simulink model "PannelTest"  (R2022b)
settings: Solver=FixedStepAuto  StartTime=0.0  StopTime=102  FixedStep=0.001  RelTol=1e-3
model workspace (MAT data in the model file):
  Manual_Auto : Simulink.Parameter (value not decoded)
  Pattern : Simulink.Parameter (value not decoded)
  Pause_Start : Simulink.Parameter (value not decoded)
  Stop : Simulink.Parameter (value not decoded)
  Unlock_Lock : Simulink.Parameter (value not decoded)
undefined symbols (not defined in the file or in its folder): DiscIntNeverNeededParam
(part 2 of 3)

== system PannelTest/PanelController/Display_State_4_Enable/Subsystem ==
  Case : Inport
  Case Default : Inport  Port=2
  Constant : Constant
  Constant1 : Constant  Value=0
  Constant2 : Constant  Value=TaskIndex
  Merge : Merge
  Switch Case Action Subsystem : Subsystem  TreatAsAtomicUnit=on
  Switch Case Action Subsystem1 : Subsystem  TreatAsAtomicUnit=on
  Enable : Outport
  FinishIndex : Outport  Port=2
  wires:
  Constant/1 -> Switch Case Action Subsystem/1(In1)
  Case/1 -> Switch Case Action Subsystem/Action
  Switch Case Action Subsystem/1(Out1) -> Merge/1
  Merge/1 -> Enable/1
  Case Default/1 -> Switch Case Action Subsystem1/Action
  Constant1/1 -> Switch Case Action Subsystem1/1(In1)
  Switch Case Action Subsystem1/1(Default) -> Merge/2
  Constant2/1 -> FinishIndex/1

== system PannelTest/PanelController/LLTaskControl_State_1_Enable/Subsystem ==
  Case : Inport
  Case Default : Inport  Port=2
  Constant : Constant
  Constant1 : Constant  Value=0
  Constant2 : Constant  Value=TaskIndex
  Merge : Merge
  Switch Case Action Subsystem : Subsystem  TreatAsAtomicUnit=on
  Switch Case Action Subsystem1 : Subsystem  TreatAsAtomicUnit=on
  Enable : Outport
  FinishIndex : Outport  Port=2
  wires:
  Constant/1 -> Switch Case Action Subsystem/1(In1)
  Case/1 -> Switch Case Action Subsystem/Action
  Switch Case Action Subsystem/1(Out1) -> Merge/1
  Merge/1 -> Enable/1
  Case Default/1 -> Switch Case Action Subsystem1/Action
  Constant1/1 -> Switch Case Action Subsystem1/1(In1)
  Switch Case Action Subsystem1/1(Default) -> Merge/2
  Constant2/1 -> FinishIndex/1

== system PannelTest/PanelController/LLTaskControl_State_2_Enable/Subsystem ==
  Case : Inport
  Case Default : Inport  Port=2
  Constant : Constant
  Constant1 : Constant  Value=0
  Constant2 : Constant  Value=TaskIndex
  Merge : Merge
  Switch Case Action Subsystem : Subsystem  TreatAsAtomicUnit=on
  Switch Case Action Subsystem1 : Subsystem  TreatAsAtomicUnit=on
  Enable : Outport
  FinishIndex : Outport  Port=2
  wires:
  Constant/1 -> Switch Case Action Subsystem/1(In1)
  Case/1 -> Switch Case Action Subsystem/Action
  Switch Case Action Subsystem/1(Out1) -> Merge/1
  Merge/1 -> Enable/1
  Case Default/1 -> Switch Case Action Subsystem1/Action
  Constant1/1 -> Switch Case Action Subsystem1/1(In1)
  Switch Case Action Subsystem1/1(Default) -> Merge/2
  Constant2/1 -> FinishIndex/1

== system PannelTest/PanelController/LLTaskControl_State_3_Enable/Subsystem ==
  Case : Inport
  Case Default : Inport  Port=2
  Constant : Constant
  Constant1 : Constant  Value=0
  Constant2 : Constant  Value=TaskIndex
  Merge : Merge
  Switch Case Action Subsystem : Subsystem  TreatAsAtomicUnit=on
  Switch Case Action Subsystem1 : Subsystem  TreatAsAtomicUnit=on
  Enable : Outport
  FinishIndex : Outport  Port=2
  wires:
  Constant/1 -> Switch Case Action Subsystem/1(In1)
  Case/1 -> Switch Case Action Subsystem/Action
  Switch Case Action Subsystem/1(Out1) -> Merge/1
  Merge/1 -> Enable/1
  Case Default/1 -> Switch Case Action Subsystem1/Action
  Constant1/1 -> Switch Case Action Subsystem1/1(In1)
  Switch Case Action Subsystem1/1(Default) -> Merge/2
  Constant2/1 -> FinishIndex/1

== system PannelTest/PanelController/LLTaskControl_State_4_Enable/Subsystem ==
  Case : Inport
  Case Default : Inport  Port=2
  Constant : Constant
  Constant1 : Constant  Value=0
  Constant2 : Constant  Value=TaskIndex
  Merge : Merge
  Switch Case Action Subsystem : Subsystem  TreatAsAtomicUnit=on
  Switch Case Action Subsystem1 : Subsystem  TreatAsAtomicUnit=on
  Enable : Outport
  FinishIndex : Outport  Port=2
  wires:
  Constant/1 -> Switch Case Action Subsystem/1(In1)
  Case/1 -> Switch Case Action Subsystem/Action
  Switch Case Action Subsystem/1(Out1) -> Merge/1
  Merge/1 -> Enable/1
  Case Default/1 -> Switch Case Action Subsystem1/Action
  Constant1/1 -> Switch Case Action Subsystem1/1(In1)
  Switch Case Action Subsystem1/1(Default) -> Merge/2
  Constant2/1 -> FinishIndex/1

== system PannelTest/PanelController/LLTaskControl_State_5_Enable/Subsystem ==
  Case : Inport
  Case Default : Inport  Port=2
  Constant : Constant
  Constant1 : Constant  Value=0
  Constant2 : Constant  Value=TaskIndex
  Merge : Merge
  Switch Case Action Subsystem : Subsystem  TreatAsAtomicUnit=on
  Switch Case Action Subsystem1 : Subsystem  TreatAsAtomicUnit=on
  Enable : Outport
  FinishIndex : Outport  Port=2
  wires:
  Constant/1 -> Switch Case Action Subsystem/1(In1)
  Case/1 -> Switch Case Action Subsystem/Action
  Switch Case Action Subsystem/1(Out1) -> Merge/1
  Merge/1 -> Enable/1
  Case Default/1 -> Switch Case Action Subsystem1/Action
  Constant1/1 -> Switch Case Action Subsystem1/1(In1)
  Switch Case Action Subsystem1/1(Default) -> Merge/2
  Constant2/1 -> FinishIndex/1

== system PannelTest/PanelController/LLTaskControl_State_6_Enable/Subsystem ==
  Case : Inport
  Case Default : Inport  Port=2
  Constant : Constant
  Constant1 : Constant  Value=0
  Constant2 : Constant  Value=TaskIndex
  Merge : Merge
  Switch Case Action Subsystem : Subsystem  TreatAsAtomicUnit=on
  Switch Case Action Subsystem1 : Subsystem  TreatAsAtomicUnit=on
  Enable : Outport
  FinishIndex : Outport  Port=2
  wires:
  Constant/1 -> Switch Case Action Subsystem/1(In1)
  Case/1 -> Switch Case Action Subsystem/Action
  Switch Case Action Subsystem/1(Out1) -> Merge/1
  Merge/1 -> Enable/1
  Case Default/1 -> Switch Case Action Subsystem1/Action
  Constant1/1 -> Switch Case Action Subsystem1/1(In1)
  Switch Case Action Subsystem1/1(Default) -> Merge/2
  Constant2/1 -> FinishIndex/1

== system PannelTest/PanelController/LLTaskControl_State_7_Enable/Subsystem ==
  Case : Inport
  Case Default : Inport  Port=2
  Constant : Constant
  Constant1 : Constant  Value=0
  Constant2 : Constant  Value=TaskIndex
  Merge : Merge
  Switch Case Action Subsystem : Subsystem  TreatAsAtomicUnit=on
  Switch Case Action Subsystem1 : Subsystem  TreatAsAtomicUnit=on
  Enable : Outport
  FinishIndex : Outport  Port=2
  wires:
  Constant/1 -> Switch Case Action Subsystem/1(In1)
  Case/1 -> Switch Case Action Subsystem/Action
  Switch Case Action Subsystem/1(Out1) -> Merge/1
  Merge/1 -> Enable/1
  Case Default/1 -> Switch Case Action Subsystem1/Action
  Constant1/1 -> Switch Case Action Subsystem1/1(In1)
  Switch Case Action Subsystem1/1(Default) -> Merge/2
  Constant2/1 -> FinishIndex/1

== system PannelTest/PanelController/LLTaskControl_State_8_Enable/Subsystem ==
  Case : Inport
  Case Default : Inport  Port=2
  Constant : Constant
  Constant1 : Constant  Value=0
  Constant2 : Constant  Value=TaskIndex
  Merge : Merge
  Switch Case Action Subsystem : Subsystem  TreatAsAtomicUnit=on
  Switch Case Action Subsystem1 : Subsystem  TreatAsAtomicUnit=on
  Enable : Outport
  FinishIndex : Outport  Port=2
  wires:
  Constant/1 -> Switch Case Action Subsystem/1(In1)
  Case/1 -> Switch Case Action Subsystem/Action
  Switch Case Action Subsystem/1(Out1) -> Merge/1
  Merge/1 -> Enable/1
  Case Default/1 -> Switch Case Action Subsystem1/Action
  Constant1/1 -> Switch Case Action Subsystem1/1(In1)
  Switch Case Action Subsystem1/1(Default) -> Merge/2
  Constant2/1 -> FinishIndex/1

== system PannelTest/PanelController/LLTaskControl_State_9_Enable/Subsystem ==
  Case : Inport
  Case Default : Inport  Port=2
  Constant : Constant
  Constant1 : Constant  Value=0
  Constant2 : Constant  Value=TaskIndex
  Merge : Merge
  Switch Case Action Subsystem : Subsystem  TreatAsAtomicUnit=on
  Switch Case Action Subsystem1 : Subsystem  TreatAsAtomicUnit=on
  Enable : Outport
  FinishIndex : Outport  Port=2
  wires:
  Constant/1 -> Switch Case Action Subsystem/1(In1)
  Case/1 -> Switch Case Action Subsystem/Action
  Switch Case Action Subsystem/1(Out1) -> Merge/1
  Merge/1 -> Enable/1
  Case Default/1 -> Switch Case Action Subsystem1/Action
  Constant1/1 -> Switch Case Action Subsystem1/1(In1)
  Switch Case Action Subsystem1/1(Default) -> Merge/2
  Constant2/1 -> FinishIndex/1

== system PannelTest/PanelController/ULTaskControl_State_1_Enable/Subsystem ==
  Case : Inport
  Case Default : Inport  Port=2
  Constant : Constant
  Constant1 : Constant  Value=0
  Constant2 : Constant  Value=TaskIndex
  Merge : Merge
  Switch Case Action Subsystem : Subsystem  TreatAsAtomicUnit=on
  Switch Case Action Subsystem1 : Subsystem  TreatAsAtomicUnit=on
  Enable : Outport
  FinishIndex : Outport  Port=2
  wires:
  Constant/1 -> Switch Case Action Subsystem/1(In1)
  Case/1 -> Switch Case Action Subsystem/Action
  Switch Case Action Subsystem/1(Out1) -> Merge/1
  Merge/1 -> Enable/1
  Case Default/1 -> Switch Case Action Subsystem1/Action
  Constant1/1 -> Switch Case Action Subsystem1/1(In1)
  Switch Case Action Subsystem1/1(Default) -> Merge/2
  Constant2/1 -> FinishIndex/1

== system PannelTest/PanelController/ULTaskControl_State_2_Enable/Subsystem ==
  Case : Inport
  Case Default : Inport  Port=2
  Constant : Constant
  Constant1 : Constant  Value=0
  Constant2 : Constant  Value=TaskIndex
  Merge : Merge
  Switch Case Action Subsystem : Subsystem  TreatAsAtomicUnit=on
  Switch Case Action Subsystem1 : Subsystem  TreatAsAtomicUnit=on
  Enable : Outport
  FinishIndex : Outport  Port=2
  wires:
  Constant/1 -> Switch Case Action Subsystem/1(In1)
  Case/1 -> Switch Case Action Subsystem/Action
  Switch Case Action Subsystem/1(Out1) -> Merge/1
  Merge/1 -> Enable/1
  Case Default/1 -> Switch Case Action Subsystem1/Action
  Constant1/1 -> Switch Case Action Subsystem1/1(In1)
  Switch Case Action Subsystem1/1(Default) -> Merge/2
  Constant2/1 -> FinishIndex/1

== system PannelTest/Tasks/LLBAutoTask/If Action Subsystem12 ==
  In1 : Inport
  Action Port : ActionPort  ActionPortLabel=if((u1 > 4))
  Out1 : Outport
  wires:
  In1/1 -> Out1/1

== system PannelTest/Tasks/LLBAutoTask/If Action Subsystem13 ==
  In1 : Inport
  Action Port : ActionPort  ActionPortLabel=else
  Out1 : Outport
  wires:
  In1/1 -> Out1/1

== system PannelTest/Tasks/LLBManualTask/If Action Subsystem12 ==
  In1 : Inport
  Action Port : ActionPort  ActionPortLabel=if((u1 > 4))
  Out1 : Outport
  wires:
  In1/1 -> Out1/1

== system PannelTest/Tasks/LLBManualTask/If Action Subsystem13 ==
  In1 : Inport
  Action Port : ActionPort  ActionPortLabel=else
  Out1 : Outport
  wires:
  In1/1 -> Out1/1

== system PannelTest/Tasks/LLFKAutoTask/If Action Subsystem12 ==
  In1 : Inport
  Action Port : ActionPort  ActionPortLabel=if((u1 > 4))
  Out1 : Outport
  wires:
  In1/1 -> Out1/1

== system PannelTest/Tasks/LLFKAutoTask/If Action Subsystem13 ==
  In1 : Inport
  Action Port : ActionPort  ActionPortLabel=else
  Out1 : Outport
  wires:
  In1/1 -> Out1/1

== system PannelTest/Tasks/LLFKManualTask/If Action Subsystem12 ==
  In1 : Inport
  Action Port : ActionPort  ActionPortLabel=if((u1 > 4))
  Out1 : Outport
  wires:
  In1/1 -> Out1/1

== system PannelTest/Tasks/LLFKManualTask/If Action Subsystem13 ==
  In1 : Inport
  Action Port : ActionPort  ActionPortLabel=else
  Out1 : Outport
  wires:
  In1/1 -> Out1/1

== system PannelTest/Tasks/LLFTask/If Action Subsystem12 ==
  In1 : Inport
  Action Port : ActionPort  ActionPortLabel=if((u1 > 4))
  Out1 : Outport
  wires:
  In1/1 -> Out1/1

== system PannelTest/Tasks/LLFTask/If Action Subsystem13 ==
  In1 : Inport
  Action Port : ActionPort  ActionPortLabel=else
  Out1 : Outport
  wires:
  In1/1 -> Out1/1

== system PannelTest/Tasks/LLWAutoTask/If Action Subsystem12 ==
  In1 : Inport
  Action Port : ActionPort  ActionPortLabel=if((u1 > 4))
  Out1 : Outport
  wires:
  In1/1 -> Out1/1

== system PannelTest/Tasks/LLWAutoTask/If Action Subsystem13 ==
  In1 : Inport
  Action Port : ActionPort  ActionPortLabel=else
  Out1 : Outport
  wires:
  In1/1 -> Out1/1

== system PannelTest/Tasks/LLWManualTask/If Action Subsystem12 ==
  In1 : Inport
  Action Port : ActionPort  ActionPortLabel=if((u1 > 4))
  Out1 : Outport
  wires:
  In1/1 -> Out1/1

== system PannelTest/Tasks/LLWManualTask/If Action Subsystem13 ==
  In1 : Inport
  Action Port : ActionPort  ActionPortLabel=else
  Out1 : Outport
  wires:
  In1/1 -> Out1/1

== system PannelTest/Tasks/PauseTask/If Action Subsystem12 ==
  In1 : Inport
  Action Port : ActionPort  ActionPortLabel=if((u1 > 4))
  Out1 : Outport
  wires:
  In1/1 -> Out1/1

== system PannelTest/Tasks/PauseTask/If Action Subsystem13 ==
  In1 : Inport
  Action Port : ActionPort  ActionPortLabel=else
  Out1 : Outport
  wires:
  In1/1 -> Out1/1

== system PannelTest/Tasks/StopTask/If Action Subsystem10 ==
  y : Inport
  Action Port : ActionPort  ActionPortLabel=if(u1 < -0)
  Out1 : Outport
  wires:
  y/1 -> Out1/1

== system PannelTest/Tasks/StopTask/If Action Subsystem11 ==
  y : Inport
  Action Port : ActionPort  ActionPortLabel=else
  Out1 : Outport
  wires:
  y/1 -> Out1/1

== system PannelTest/Tasks/StopTask/If Action Subsystem12 ==
  In1 : Inport
  Action Port : ActionPort  ActionPortLabel=if((u1 > 4))
  Out1 : Outport
  wires:
  In1/1 -> Out1/1

== system PannelTest/Tasks/StopTask/If Action Subsystem13 ==
  In1 : Inport
  Action Port : ActionPort  ActionPortLabel=else
  Out1 : Outport
  wires:
  In1/1 -> Out1/1

== system PannelTest/Tasks/StopTask/If Action Subsystem4 ==
  In1 : Inport
  Action Port : ActionPort  ActionPortLabel=if((u1 <= 1))
  Out1 : Outport
  wires:
  In1/1 -> Out1/1

== system PannelTest/Tasks/StopTask/If Action Subsystem5 ==
  In1 : Inport
  Action Port : ActionPort  ActionPortLabel=else
  Out1 : Outport
  wires:
  In1/1 -> Out1/1

== system PannelTest/Tasks/StopTask/If Action Subsystem6 ==
  In1 : Inport
  Action Port : ActionPort  ActionPortLabel=if((u1 <= 1))
  Out1 : Outport
  wires:
  In1/1 -> Out1/1

== system PannelTest/Tasks/StopTask/If Action Subsystem7 ==
  In1 : Inport
  Action Port : ActionPort  ActionPortLabel=else
  Out1 : Outport
  wires:
  In1/1 -> Out1/1

== system PannelTest/Tasks/StopTask/If Action Subsystem8 ==
  y : Inport
  Action Port : ActionPort  ActionPortLabel=if(u1 < -0)
  Out1 : Outport
  wires:
  y/1 -> Out1/1

== system PannelTest/Tasks/StopTask/If Action Subsystem9 ==
  In1 : Inport
  Action Port : ActionPort  ActionPortLabel=else
  Out1 : Outport
  wires:
  In1/1 -> Out1/1

== system PannelTest/Tasks/ULLockTask/If Action Subsystem12 ==
  In1 : Inport
  Action Port : ActionPort  ActionPortLabel=if((u1 > 4))
  Out1 : Outport
  wires:
  In1/1 -> Out1/1

== system PannelTest/Tasks/ULLockTask/If Action Subsystem13 ==
  In1 : Inport
  Action Port : ActionPort  ActionPortLabel=else
  Out1 : Outport
  wires:
  In1/1 -> Out1/1

== system PannelTest/Tasks/ULUnLockTask/If Action Subsystem12 ==
  In1 : Inport
  Action Port : ActionPort  ActionPortLabel=if((u1 > 4))
  Out1 : Outport
  wires:
  In1/1 -> Out1/1

== system PannelTest/Tasks/ULUnLockTask/If Action Subsystem13 ==
  In1 : Inport
  Action Port : ActionPort  ActionPortLabel=else
  Out1 : Outport
  wires:
  In1/1 -> Out1/1

== system PannelTest/PanelController/Display_State_1_Enable/Subsystem/Switch Case Action Subsystem ==
  In1 : Inport
  Action Port : ActionPort  ActionPortLabel=case [ 1 ]:
  Out1 : Outport
  wires:
  In1/1 -> Out1/1

== system PannelTest/PanelController/Display_State_1_Enable/Subsystem/Switch Case Action Subsystem1 ==
  In1 : Inport
  Action Port : ActionPort  ActionPortLabel=default:
  Default : Outport
  wires:
  In1/1 -> Default/1

== system PannelTest/PanelController/Display_State_2_Enable/Subsystem/Switch Case Action Subsystem ==
  In1 : Inport
  Action Port : ActionPort  ActionPortLabel=case [ 2 ]:
  Out1 : Outport
  wires:
  In1/1 -> Out1/1

== system PannelTest/PanelController/Display_State_2_Enable/Subsystem/Switch Case Action Subsystem1 ==
  In1 : Inport
  Action Port : ActionPort  ActionPortLabel=default:
  Default : Outport
  wires:
  In1/1 -> Default/1

== system PannelTest/PanelController/Display_State_3_Enable/Subsystem/Switch Case Action Subsystem ==
  In1 : Inport
  Action Port : ActionPort  ActionPortLabel=case [ 3 ]:
  Out1 : Outport
  wires:
  In1/1 -> Out1/1

== system PannelTest/PanelController/Display_State_3_Enable/Subsystem/Switch Case Action Subsystem1 ==
  In1 : Inport
  Action Port : ActionPort  ActionPortLabel=default:
  Default : Outport
  wires:
  In1/1 -> Default/1

== system PannelTest/PanelController/Display_State_4_Enable/Subsystem/Switch Case Action Subsystem ==
  In1 : Inport
  Action Port : ActionPort  ActionPortLabel=case [ 4 ]:
  Out1 : Outport
  wires:
  In1/1 -> Out1/1

== system PannelTest/PanelController/Display_State_4_Enable/Subsystem/Switch Case Action Subsystem1 ==
  In1 : Inport
  Action Port : ActionPort  ActionPortLabel=default:
  Default : Outport
  wires:
  In1/1 -> Default/1

== system PannelTest/PanelController/LLTaskControl_State_1_Enable/Subsystem/Switch Case Action Subsystem ==
  In1 : Inport
  Action Port : ActionPort  ActionPortLabel=case [ 1 ]:
  Out1 : Outport
  wires:
  In1/1 -> Out1/1

== system PannelTest/PanelController/LLTaskControl_State_1_Enable/Subsystem/Switch Case Action Subsystem1 ==
  In1 : Inport
  Action Port : ActionPort  ActionPortLabel=default:
  Default : Outport
  wires:
  In1/1 -> Default/1

== system PannelTest/PanelController/LLTaskControl_State_2_Enable/Subsystem/Switch Case Action Subsystem ==
  In1 : Inport
  Action Port : ActionPort  ActionPortLabel=case [ 2 ]:
  Out1 : Outport
  wires:
  In1/1 -> Out1/1

== system PannelTest/PanelController/LLTaskControl_State_2_Enable/Subsystem/Switch Case Action Subsystem1 ==
  In1 : Inport
  Action Port : ActionPort  ActionPortLabel=default:
  Default : Outport
  wires:
  In1/1 -> Default/1

== system PannelTest/PanelController/LLTaskControl_State_3_Enable/Subsystem/Switch Case Action Subsystem ==
  In1 : Inport
  Action Port : ActionPort  ActionPortLabel=case [ 3 ]:
  Out1 : Outport
  wires:
  In1/1 -> Out1/1

== system PannelTest/PanelController/LLTaskControl_State_3_Enable/Subsystem/Switch Case Action Subsystem1 ==
  In1 : Inport
  Action Port : ActionPort  ActionPortLabel=default:
  Default : Outport
  wires:
  In1/1 -> Default/1

== system PannelTest/PanelController/LLTaskControl_State_4_Enable/Subsystem/Switch Case Action Subsystem ==
  In1 : Inport
  Action Port : ActionPort  ActionPortLabel=case [ 4 ]:
  Out1 : Outport
  wires:
  In1/1 -> Out1/1

== system PannelTest/PanelController/LLTaskControl_State_4_Enable/Subsystem/Switch Case Action Subsystem1 ==
  In1 : Inport
  Action Port : ActionPort  ActionPortLabel=default:
  Default : Outport
  wires:
  In1/1 -> Default/1

== system PannelTest/PanelController/LLTaskControl_State_5_Enable/Subsystem/Switch Case Action Subsystem ==
  In1 : Inport
  Action Port : ActionPort  ActionPortLabel=case [ 5 ]:
  Out1 : Outport
  wires:
  In1/1 -> Out1/1

== system PannelTest/PanelController/LLTaskControl_State_5_Enable/Subsystem/Switch Case Action Subsystem1 ==
  In1 : Inport
  Action Port : ActionPort  ActionPortLabel=default:
  Default : Outport
  wires:
  In1/1 -> Default/1

== system PannelTest/PanelController/LLTaskControl_State_6_Enable/Subsystem/Switch Case Action Subsystem ==
  In1 : Inport
  Action Port : ActionPort  ActionPortLabel=case [ 6 ]:
  Out1 : Outport
  wires:
  In1/1 -> Out1/1

== system PannelTest/PanelController/LLTaskControl_State_6_Enable/Subsystem/Switch Case Action Subsystem1 ==
  In1 : Inport
  Action Port : ActionPort  ActionPortLabel=default:
  Default : Outport
  wires:
  In1/1 -> Default/1

== system PannelTest/PanelController/LLTaskControl_State_7_Enable/Subsystem/Switch Case Action Subsystem ==
  In1 : Inport
  Action Port : ActionPort  ActionPortLabel=case [ 7 ]:
  Out1 : Outport
  wires:
  In1/1 -> Out1/1

== system PannelTest/PanelController/LLTaskControl_State_7_Enable/Subsystem/Switch Case Action Subsystem1 ==
  In1 : Inport
  Action Port : ActionPort  ActionPortLabel=default:
  Default : Outport
  wires:
  In1/1 -> Default/1

== system PannelTest/PanelController/LLTaskControl_State_8_Enable/Subsystem/Switch Case Action Subsystem ==
  In1 : Inport
  Action Port : ActionPort  ActionPortLabel=case [ 8 ]:
  Out1 : Outport
  wires:
  In1/1 -> Out1/1

== system PannelTest/PanelController/LLTaskControl_State_8_Enable/Subsystem/Switch Case Action Subsystem1 ==
  In1 : Inport
  Action Port : ActionPort  ActionPortLabel=default:
  Default : Outport
  wires:
  In1/1 -> Default/1

== system PannelTest/PanelController/LLTaskControl_State_9_Enable/Subsystem/Switch Case Action Subsystem ==
  In1 : Inport
  Action Port : ActionPort  ActionPortLabel=case [ 9 ]:
  Out1 : Outport
  wires:
  In1/1 -> Out1/1

== system PannelTest/PanelController/LLTaskControl_State_9_Enable/Subsystem/Switch Case Action Subsystem1 ==
  In1 : Inport
  Action Port : ActionPort  ActionPortLabel=default:
  Default : Outport
  wires:
  In1/1 -> Default/1

== system PannelTest/PanelController/ULTaskControl_State_1_Enable/Subsystem/Switch Case Action Subsystem ==
  In1 : Inport
  Action Port : ActionPort  ActionPortLabel=case [ 1 ]:
  Out1 : Outport
  wires:
  In1/1 -> Out1/1

== system PannelTest/PanelController/ULTaskControl_State_1_Enable/Subsystem/Switch Case Action Subsystem1 ==
  In1 : Inport
  Action Port : ActionPort  ActionPortLabel=default:
  Default : Outport
  wires:
  In1/1 -> Default/1

== system PannelTest/PanelController/ULTaskControl_State_2_Enable/Subsystem/Switch Case Action Subsystem ==
  In1 : Inport
  Action Port : ActionPort  ActionPortLabel=case [ 2 ]:
  Out1 : Outport
  wires:
  In1/1 -> Out1/1

== system PannelTest/PanelController/ULTaskControl_State_2_Enable/Subsystem/Switch Case Action Subsystem1 ==
  In1 : Inport
  Action Port : ActionPort  ActionPortLabel=default:
  Default : Outport
  wires:
  In1/1 -> Default/1

== stateflow chart PannelTest/PanelController/LowerLimbTaskControlStateMachine ==
  state PauseTask
    ControlState = 9;
  state StopTask
    ControlState = 1;
  state StartTask
    state Start
    state LLFTask
      ControlState = 2;
    state LLFK
      state LLFK
      state LLFKManualTask
        ControlState = 3;
      state LLFKAutoTask
        ControlState = 4;
      (default) -> StartTask.LLFK.LLFK
      StartTask.LLFK.LLFK -> LLFKManualTask [order 1] : [ManualAuto~="LLFK_Auto"]
      StartTask.LLFK.LLFK -> LLFKAutoTask [order 2] : [ManualAuto=="LLFK_Auto"]
      LLFKManualTask -> StartTask.LLFK.LLFK : [ManualAuto=="LLFK_Auto"]
      LLFKAutoTask -> StartTask.LLFK.LLFK : [ManualAuto~="LLFK_Auto"]
    state LLB
      state LLB
      state LLBManualTask
        ControlState = 5;
      state LLBAutoTask
        ControlState = 6;
      (default) -> StartTask.LLB.LLB
      StartTask.LLB.LLB -> LLBAutoTask [order 2] : [ManualAuto=="LLB_Auto"]
      StartTask.LLB.LLB -> LLBManualTask [order 1] : [ManualAuto~="LLB_Auto"]
      LLBAutoTask -> StartTask.LLB.LLB : [ManualAuto~="LLB_Auto"]
      LLBManualTask -> StartTask.LLB.LLB : [ManualAuto=="LLB_Auto"]
    state LLW
      state LLW
      state LLWManualTask
        ControlState = 7;
      state LLWAutoTask
        ControlState = 8;
      (default) -> StartTask.LLW.LLW
      StartTask.LLW.LLW -> LLWManualTask [order 1] : [ManualAuto~="LLW_Auto"]
      StartTask.LLW.LLW -> LLWAutoTask [order 2] : [ManualAuto=="LLW_Auto"]
      LLWAutoTask -> StartTask.LLW.LLW : [ManualAuto~="LLW_Auto"]
      LLWManualTask -> StartTask.LLW.LLW : [ManualAuto=="LLW_Auto"]
    (default) -> Start
    Start -> LLFTask [order 1] : [Mode=="Lower_Limb_Follow"]
    Start -> StartTask.LLFK [order 2] : [Mode=="Lower_Limb_FlutterKick"]
    Start -> StartTask.LLW [order 4] : [Mode=="Lower_Limb_Walk"]
    StartTask.LLB -> Start : [Mode~="Lower_Limb_Breaststroke"]
    LLFTask -> Start : [Mode~="Lower_Limb_Follow"]
    StartTask.LLFK -> Start : [Mode~="Lower_Limb_FlutterKick"]
    StartTask.LLW -> Start : [Mode~="Lower_Limb_Walk"]
    Start -> StartTask.LLB [order 3] : [Mode=="Lower_Limb_Breaststroke"]
  (default) -> PauseTask
  PauseTask -> StartTask [order 2] : [State=="Start"]
  PauseTask -> StopTask [order 1] : [State=="Stop"]
  StartTask -> PauseTask : [State=="Pause"]
  StopTask -> StartTask : [State=="Start"]
  data: State input; Mode input; ManualAuto input; ControlState output; TaskFinished input

== matlab function PannelTest/Tasks/StopTask/MATLAB Function1 ==
  data: u input; y output; Pos input
function y = Current_P(u, Pos)
y = sign(u)*min(abs(u),abs(Pos)*0.1);

== stateflow chart PannelTest/PanelController/KnobStateMachine ==
  state Start
    kState = "Start";
  state Adjust
    state LLF_Adjust
    state Adjust
      kState = "Adjust";
    state LLFK_Adjust
      state LLFK_Auto
      state LLFK_Adjust
        kState = "LLFK_Adjust";
      state LLFK_Freq_Adjust
        state LLFK_Freq_Adjust
          kState = "LLFK_Freq";
          LLFK_Freq = 0;
          LLFK_Torque_Up = 0;
          LLFK_Torque_Down = 0;
          LLFK_Pos_Up = 0;
          LLFK_Pos_Down = 0;
          LLB_Freq = 0;
          LLB_Torque_Up = 0;
          LLB_Torque_Down = 0;
          LLB_Pos_Up = 0;
          LLB_Pos_Down = 0;
          LLW_Freq = 0;
          LLW_Torque_Up = 0;
          LLW_Torque_Down = 0;
          LLW_Pos_Up = 0;
          LLW_Pos_Down = 0;
          Freq_Up_temp = 0;
          Freq_Down_temp = 0;
        state Freq_Up
          if(Freq_Up==0)
          Freq_Up_temp = 0;
          LLFK_Freq = 1;
          end
        state Freq_Down
          if(Freq_Down==0)
          Freq_Down_temp = 0;
          LLFK_Freq = -1;
          end
        (default) -> Adjust.LLFK_Adjust.LLFK_Freq_Adjust.LLFK_Freq_Adjust
        Adjust.LLFK_Adjust.LLFK_Freq_Adjust.LLFK_Freq_Adjust -> Adjust.LLFK_Adjust.LLFK_Freq_Adjust.Freq_Down [order 2] : [(Freq_Down_temp==0)&&(Freq_Down>0)]{Freq_Down_temp=1;}
        Adjust.LLFK_Adjust.LLFK_Freq_Adjust.LLFK_Freq_Adjust -> Adjust.LLFK_Adjust.LLFK_Freq_Adjust.Freq_Up [order 1] : [(Freq_Up_temp==0)&&(Freq_Up>0)]{Freq_Up_temp=1;}
        Adjust.LLFK_Adjust.LLFK_Freq_Adjust.Freq_Up -> Adjust.LLFK_Adjust.LLFK_Freq_Adjust.LLFK_Freq_Adjust : [Freq_Up_temp == 0]
        Adjust.LLFK_Adjust.LLFK_Freq_Adjust.Freq_Down -> Adjust.LLFK_Adjust.LLFK_Freq_Adjust.LLFK_Freq_Adjust : [Freq_Down_temp == 0]
      state LLFK_Torque_Adjust
        state Negtive_Up
          if(Negtive_Up==0)
          Negtive_Up_temp = 0;
          LLFK_Torque_Down = 1;
          end
        state LLFK_Torque_Adjust
          kState = "LLFK_Torq";
          LLFK_Freq = 0;
          LLFK_Torque_Up = 0;
          LLFK_Torque_Down = 0;
          LLFK_Pos_Up = 0;
          LLFK_Pos_Down = 0;
          LLB_Freq = 0;
          LLB_Torque_Up = 0;
          LLB_Torque_Down = 0;
          LLB_Pos_Up = 0;
          LLB_Pos_Down = 0;
          LLW_Freq = 0;
          LLW_Torque_Up = 0;
          LLW_Torque_Down = 0;
          LLW_Pos_Up = 0;
          LLW_Pos_Down = 0;
          Negtive_Up_temp = 0;
          Negtive_Down_temp = 0;
          Positive_Up_temp = 0;
          Positive_Down_temp = 0;
        state Negtive_Down
          if(Negtive_Down==0)
          Negtive_Down_temp = 0;
          LLFK_Torque_Down = -1;
          end
        state Positive_Up
          if(Positive_Up==0)
          Positive_Up_temp = 0;
          LLFK_Torque_Up = 1;
          end
        state Positive_Down
          if(Positive_Down==0)
          Positive_Down_temp = 0;
          LLFK_Torque_Up = -1;
          end
        (default) -> Adjust.LLFK_Adjust.LLFK_Torque_Adjust.LLFK_Torque_Adjust
        Adjust.LLFK_Adjust.LLFK_Torque_Adjust.LLFK_Torque_Adjust -> Adjust.LLFK_Adjust.LLFK_Torque_Adjust.Negtive_Up [order 4] : [(Negtive_Up_temp==0)&&(Negtive_Up>0)]{Negtive_Up_temp=1;}
        Adjust.LLFK_Adjust.LLFK_Torque_Adjust.LLFK_Torque_Adjust -> Adjust.LLFK_Adjust.LLFK_Torque_Adjust.Negtive_Down [order 2] : [(Negtive_Down_temp==0)&&(Negtive_Down>0)]{Negtive_Down_temp=1;}
        Adjust.LLFK_Adjust.LLFK_Torque_Adjust.Negtive_Down -> Adjust.LLFK_Adjust.LLFK_Torque_Adjust.LLFK_Torque_Adjust : [Negtive_Down_temp == 0]
        Adjust.LLFK_Adjust.LLFK_Torque_Adjust.Negtive_Up -> Adjust.LLFK_Adjust.LLFK_Torque_Adjust.LLFK_Torque_Adjust : [Negtive_Up_temp == 0]
        Adjust.LLFK_Adjust.LLFK_Torque_Adjust.LLFK_Torque_Adjust -> Adjust.LLFK_Adjust.LLFK_Torque_Adjust.Positive_Up [order 3] : [(Positive_Up_temp==0)&&(Positive_Up>0)]{Positive_Up_temp=1;}
        Adjust.LLFK_Adjust.LLFK_Torque_Adjust.LLFK_Torque_Adjust -> Adjust.LLFK_Adjust.LLFK_Torque_Adjust.Positive_Down [order 1] : [(Positive_Down_temp==0)&&(Positive_Down>0)]{Positive_Down_temp=1;}
        Adjust.LLFK_Adjust.LLFK_Torque_Adjust.Positive_Up -> Adjust.LLFK_Adjust.LLFK_Torque_Adjust.LLFK_Torque_Adjust : [Positive_Up_temp == 0]
        Adjust.LLFK_Adjust.LLFK_Torque_Adjust.Positive_Down -> Adjust.LLFK_Adjust.LLFK_Torque_Adjust.LLFK_Torque_Adjust : [Positive_Down_temp == 0]
      state LLFK_Pos_Adjust
        state Negtive_Up
          if(Negtive_Up==0)
          Negtive_Up_temp = 0;
          LLFK_Pos_Down = 1;
          end
        state LLFK_Pos_Adjust
          kState = "LLFK_Pos";
          LLFK_Freq = 0;
          LLFK_Torque_Up = 0;
          LLFK_Torque_Down = 0;
          LLFK_Pos_Up = 0;
          LLFK_Pos_Down = 0;
          LLB_Freq = 0;
          LLB_Torque_Up = 0;
          LLB_Torque_Down = 0;
          LLB_Pos_Up = 0;
          LLB_Pos_Down = 0;
          LLW_Freq = 0;
          LLW_Torque_Up = 0;
          LLW_Torque_Down = 0;
          LLW_Pos_Up = 0;
          LLW_Pos_Down = 0;
          Negtive_Up_temp = 0;
          Negtive_Down_temp = 0;
          Positive_Up_temp = 0;
          Positive_Down_temp = 0;
        state Negtive_Down
          if(Negtive_Down==0)
          Negtive_Down_temp = 0;
          LLFK_Pos_Down = -1;
          end
        state Positive_Up
          if(Positive_Up==0)
          Positive_Up_temp = 0;
          LLFK_Pos_Up = 1;
          end
        state Positive_Down
          if(Positive_Down==0)
          Positive_Down_temp = 0;
          LLFK_Pos_Up = -1;
          end
        (default) -> Adjust.LLFK_Adjust.LLFK_Pos_Adjust.LLFK_Pos_Adjust
        Adjust.LLFK_Adjust.LLFK_Pos_Adjust.LLFK_Pos_Adjust -> Adjust.LLFK_Adjust.LLFK_Pos_Adjust.Negtive_Up [order 4] : [(Negtive_Up_temp==0)&&(Negtive_Up>0)]{Negtive_Up_temp=1;}
        Adjust.LLFK_Adjust.LLFK_Pos_Adjust.LLFK_Pos_Adjust -> Adjust.LLFK_Adjust.LLFK_Pos_Adjust.Negtive_Down [order 2] : [(Negtive_Down_temp==0)&&(Negtive_Down>0)]{Negtive_Down_temp=1;}
        Adjust.LLFK_Adjust.LLFK_Pos_Adjust.Negtive_Down -> Adjust.LLFK_Adjust.LLFK_Pos_Adjust.LLFK_Pos_Adjust : [Negtive_Down_temp == 0]
        Adjust.LLFK_Adjust.LLFK_Pos_Adjust.Negtive_Up -> Adjust.LLFK_Adjust.LLFK_Pos_Adjust.LLFK_Pos_Adjust : [Negtive_Up_temp == 0]
        Adjust.LLFK_Adjust.LLFK_Pos_Adjust.LLFK_Pos_Adjust -> Adjust.LLFK_Adjust.LLFK_Pos_Adjust.Positive_Up [order 3] : [(Positive_Up_temp==0)&&(Positive_Up>0)]{Positive_Up_temp=1;}
        Adjust.LLFK_Adjust.LLFK_Pos_Adjust.LLFK_Pos_Adjust -> Adjust.LLFK_Adjust.LLFK_Pos_Adjust.Positive_Down [order 1] : [(Positive_Down_temp==0)&&(Positive_Down>0)]{Positive_Down_temp=1;}
        Adjust.LLFK_Adjust.LLFK_Pos_Adjust.Positive_Up -> Adjust.LLFK_Adjust.LLFK_Pos_Adjust.LLFK_Pos_Adjust : [Positive_Up_temp == 0]
        Adjust.LLFK_Adjust.LLFK_Pos_Adjust.Positive_Down -> Adjust.LLFK_Adjust.LLFK_Pos_Adjust.LLFK_Pos_Adjust : [Positive_Down_temp == 0]
      Adjust.LLFK_Adjust.LLFK_Adjust -> LLFK_Auto [order 4] : [ManualAuto=="LLFK_Auto"]{Display_State=1;}
      LLFK_Auto -> Adjust.LLFK_Adjust.LLFK_Adjust : [ManualAuto~="LLFK_Auto"]{Display_State=2;}
      (default) -> Adjust.LLFK_Adjust.LLFK_Adjust
      Adjust.LLFK_Adjust.LLFK_Pos_Adjust -> Adjust.LLFK_Adjust.LLFK_Adjust : [ManualAuto~="LLFK_Manual_Pos"]
      Adjust.LLFK_Adjust.LLFK_Adjust -> Adjust.LLFK_Adjust.LLFK_Freq_Adjust [order 3] : [ManualAuto=="LLFK_Manual_Freq"]
      Adjust.LLFK_Adjust.LLFK_Freq_Adjust -> Adjust.LLFK_Adjust.LLFK_Adjust : [ManualAuto~="LLFK_Manual_Freq"]
      Adjust.LLFK_Adjust.LLFK_Adjust -> Adjust.LLFK_Adjust.LLFK_Pos_Adjust [order 1] : [ManualAuto=="LLFK_Manual_Pos"]
      Adjust.LLFK_Adjust.LLFK_Adjust -> Adjust.LLFK_Adjust.LLFK_Torque_Adjust [order 2] : [ManualAuto=="LLFK_Manual_Torque"]
      Adjust.LLFK_Adjust.LLFK_Torque_Adjust -> Adjust.LLFK_Adjust.LLFK_Adjust : [ManualAuto~="LLFK_Manual_Torque"]
    state LLB_Adjust
      state LLB_Auto
      state LLB_Adjust
        kState = "LLB_Adjust";
      state LLB_Freq_Adjust
        state LLB_Freq_Adjust
          kState = "LLB_Freq";
          LLFK_Freq = 0;
          LLFK_Torque_Up = 0;
          LLFK_Torque_Down = 0;
          LLFK_Pos_Up = 0;
          LLFK_Pos_Down = 0;
          LLB_Freq = 0;
          LLB_Torque_Up = 0;
          LLB_Torque_Down = 0;
          LLB_Pos_Up = 0;
          LLB_Pos_Down = 0;
          LLW_Freq = 0;
          LLW_Torque_Up = 0;
          LLW_Torque_Down = 0;
          LLW_Pos_Up = 0;
          LLW_Pos_Down = 0;
          Freq_Up_temp = 0;
          Freq_Down_temp = 0;
        state Freq_Up
          if(Freq_Up==0)
          Freq_Up_temp = 0;
          LLB_Freq = 1;
          end
        state Freq_Down
          if(Freq_Down==0)
          Freq_Down_temp = 0;
          LLB_Freq = -1;
          end
        (default) -> Adjust.LLB_Adjust.LLB_Freq_Adjust.LLB_Freq_Adjust
        Adjust.LLB_Adjust.LLB_Freq_Adjust.LLB_Freq_Adjust -> Adjust.LLB_Adjust.LLB_Freq_Adjust.Freq_Down [order 2] : [(Freq_Down_temp==0)&&(Freq_Down>0)]{Freq_Down_temp=1;}
        Adjust.LLB_Adjust.LLB_Freq_Adjust.LLB_Freq_Adjust -> Adjust.LLB_Adjust.LLB_Freq_Adjust.Freq_Up [order 1] : [(Freq_Up_temp==0)&&(Freq_Up>0)]{Freq_Up_temp=1;}
        Adjust.LLB_Adjust.LLB_Freq_Adjust.Freq_Up -> Adjust.LLB_Adjust.LLB_Freq_Adjust.LLB_Freq_Adjust : [Freq_Up_temp == 0]
        Adjust.LLB_Adjust.LLB_Freq_Adjust.Freq_Down -> Adjust.LLB_Adjust.LLB_Freq_Adjust.LLB_Freq_Adjust : [Freq_Down_temp == 0]
      state LLB_Torque_Adjust
        state Negtive_Up
          if(Negtive_Up==0)
          Negtive_Up_temp = 0;
          LLB_Torque_Down = 1;
          end
        state LLB_Torque_Adjust
          kState = "LLB_Torq";
          LLFK_Freq = 0;
          LLFK_Torque_Up = 0;
          LLFK_Torque_Down = 0;
          LLFK_Pos_Up = 0;
          LLFK_Pos_Down = 0;
          LLB_Freq = 0;
          LLB_Torque_Up = 0;
          LLB_Torque_Down = 0;
          LLB_Pos_Up = 0;
          LLB_Pos_Down = 0;
          LLW_Freq = 0;
          LLW_Torque_Up = 0;
          LLW_Torque_Down = 0;
          LLW_Pos_Up = 0;
          LLW_Pos_Down = 0;
          Negtive_Up_temp = 0;
          Negtive_Down_temp = 0;
          Positive_Up_temp = 0;
          Positive_Down_temp = 0;
        state Negtive_Down
          if(Negtive_Down==0)
          Negtive_Down_temp = 0;
          LLB_Torque_Down = -1;
          end
        state Positive_Up
          if(Positive_Up==0)
          Positive_Up_temp = 0;
          LLB_Torque_Up = 1;
          end
        state Positive_Down
          if(Positive_Down==0)
          Positive_Down_temp = 0;
          LLB_Torque_Up = -1;
          end
        (default) -> Adjust.LLB_Adjust.LLB_Torque_Adjust.LLB_Torque_Adjust
        Adjust.LLB_Adjust.LLB_Torque_Adjust.LLB_Torque_Adjust -> Adjust.LLB_Adjust.LLB_Torque_Adjust.Negtive_Up [order 4] : [(Negtive_Up_temp==0)&&(Negtive_Up>0)]{Negtive_Up_temp=1;}
        Adjust.LLB_Adjust.LLB_Torque_Adjust.LLB_Torque_Adjust -> Adjust.LLB_Adjust.LLB_Torque_Adjust.Negtive_Down [order 2] : [(Negtive_Down_temp==0)&&(Negtive_Down>0)]{Negtive_Down_temp=1;}
        Adjust.LLB_Adjust.LLB_Torque_Adjust.Negtive_Down -> Adjust.LLB_Adjust.LLB_Torque_Adjust.LLB_Torque_Adjust : [Negtive_Down_temp == 0]
        Adjust.LLB_Adjust.LLB_Torque_Adjust.Negtive_Up -> Adjust.LLB_Adjust.LLB_Torque_Adjust.LLB_Torque_Adjust : [Negtive_Up_temp == 0]
        Adjust.LLB_Adjust.LLB_Torque_Adjust.LLB_Torque_Adjust -> Adjust.LLB_Adjust.LLB_Torque_Adjust.Positive_Down [order 1] : [(Positive_Down_temp==0)&&(Positive_Down>0)]{Positive_Down_temp=1;}
        Adjust.LLB_Adjust.LLB_Torque_Adjust.LLB_Torque_Adjust -> Adjust.LLB_Adjust.LLB_Torque_Adjust.Positive_Up [order 3] : [(Positive_Up_temp==0)&&(Positive_Up>0)]{Positive_Up_temp=1;}
        Adjust.LLB_Adjust.LLB_Torque_Adjust.Positive_Up -> Adjust.LLB_Adjust.LLB_Torque_Adjust.LLB_Torque_Adjust : [Positive_Up_temp == 0]
        Adjust.LLB_Adjust.LLB_Torque_Adjust.Positive_Down -> Adjust.LLB_Adjust.LLB_Torque_Adjust.LLB_Torque_Adjust : [Positive_Down_temp == 0]
      state LLB_Pos_Adjust
        state Negtive_Up
          if(Negtive_Up==0)
          Negtive_Up_temp = 0;
          LLB_Pos_Down = 1;
          end
        state LLB_Pos_Adjust
          kState = "LLB_Pos";
          LLFK_Freq = 0;
          LLFK_Torque_Up = 0;
          LLFK_Torque_Down = 0;
          LLFK_Pos_Up = 0;
          LLFK_Pos_Down = 0;
          LLB_Freq = 0;
          LLB_Torque_Up = 0;
          LLB_Torque_Down = 0;
          LLB_Pos_Up = 0;
          LLB_Pos_Down = 0;
          LLW_Freq = 0;
          LLW_Torque_Up = 0;
          LLW_Torque_Down = 0;
          LLW_Pos_Up = 0;
          LLW_Pos_Down = 0;
          Negtive_Up_temp = 0;
          Negtive_Down_temp = 0;
          Positive_Up_temp = 0;
          Positive_Down_temp = 0;
        state Negtive_Down
          if(Negtive_Down==0)
          Negtive_Down_temp = 0;
          LLB_Pos_Down = -1;
          end
        state Positive_Up
          if(Positive_Up==0)
          Positive_Up_temp = 0;
          LLB_Pos_Up = 1;
          end
        state Positive_Down
          if(Positive_Down==0)
          Positive_Down_temp = 0;
          LLB_Pos_Up = -1;
          end
        (default) -> Adjust.LLB_Adjust.LLB_Pos_Adjust.LLB_Pos_Adjust
        Adjust.LLB_Adjust.LLB_Pos_Adjust.LLB_Pos_Adjust -> Adjust.LLB_Adjust.LLB_Pos_Adjust.Negtive_Up [order 4] : [(Negtive_Up_temp==0)&&(Negtive_Up>0)]{Negtive_Up_temp=1;}
        Adjust.LLB_Adjust.LLB_Pos_Adjust.LLB_Pos_Adjust -> Adjust.LLB_Adjust.LLB_Pos_Adjust.Negtive_Down [order 2] : [(Negtive_Down_temp==0)&&(Negtive_Down>0)]{Negtive_Down_temp=1;}
        Adjust.LLB_Adjust.LLB_Pos_Adjust.Negtive_Down -> Adjust.LLB_Adjust.LLB_Pos_Adjust.LLB_Pos_Adjust : [Negtive_Down_temp == 0]
        Adjust.LLB_Adjust.LLB_Pos_Adjust.Negtive_Up -> Adjust.LLB_Adjust.LLB_Pos_Adjust.LLB_Pos_Adjust : [Negtive_Up_temp == 0]
        Adjust.LLB_Adjust.LLB_Pos_Adjust.LLB_Pos_Adjust -> Adjust.LLB_Adjust.LLB_Pos_Adjust.Positive_Up [order 3] : [(Positive_Up_temp==0)&&(Positive_Up>0)]{Positive_Up_temp=1;}
        Adjust.LLB_Adjust.LLB_Pos_Adjust.LLB_Pos_Adjust -> Adjust.LLB_Adjust.LLB_Pos_Adjust.Positive_Down [order 1] : [(Positive_Down_temp==0)&&(Positive_Down>0)]{Positive_Down_temp=1;}
        Adjust.LLB_Adjust.LLB_Pos_Adjust.Positive_Up -> Adjust.LLB_Adjust.LLB_Pos_Adjust.LLB_Pos_Adjust : [Positive_Up_temp == 0]
        Adjust.LLB_Adjust.LLB_Pos_Adjust.Positive_Down -> Adjust.LLB_Adjust.LLB_Pos_Adjust.LLB_Pos_Adjust : [Positive_Down_temp == 0]
      Adjust.LLB_Adjust.LLB_Adjust -> LLB_Auto [order 4] : [ManualAuto=="LLB_Auto"]{Display_State=1;}
      LLB_Auto -> Adjust.LLB_Adjust.LLB_Adjust : [ManualAuto~="LLB_Auto"]{Display_State=3;}
      (default) -> Adjust.LLB_Adjust.LLB_Adjust
      Adjust.LLB_Adjust.LLB_Pos_Adjust -> Adjust.LLB_Adjust.LLB_Adjust : [ManualAuto~="LLB_Manual_Pos"]
      Adjust.LLB_Adjust.LLB_Adjust -> Adjust.LLB_Adjust.LLB_Freq_Adjust [order 3] : [ManualAuto=="LLB_Manual_Freq"]
      Adjust.LLB_Adjust.LLB_Freq_Adjust -> Adjust.LLB_Adjust.LLB_Adjust : [ManualAuto~="LLB_Manual_Freq"]
      Adjust.LLB_Adjust.LLB_Adjust -> Adjust.LLB_Adjust.LLB_Pos_Adjust [order 1] : [ManualAuto=="LLB_Manual_Pos"]
      Adjust.LLB_Adjust.LLB_Adjust -> Adjust.LLB_Adjust.LLB_Torque_Adjust [order 2] : [ManualAuto=="LLB_Manual_Torque"]
      Adjust.LLB_Adjust.LLB_Torque_Adjust -> Adjust.LLB_Adjust.LLB_Adjust : [ManualAuto~="LLB_Manual_Torque"]
    state LLW_Adjust
      state LLW_Auto
      state LLW_Adjust
        kState = "LLW_Adjust";
      state LLW_Freq_Adjust
        state LLW_Freq_Adjust
          kState = "LLW_Freq";
          LLFK_Freq = 0;
          LLFK_Torque_Up = 0;
          LLFK_Torque_Down = 0;
          LLFK_Pos_Up = 0;
          LLFK_Pos_Down = 0;
          LLB_Freq = 0;
          LLB_Torque_Up = 0;
          LLB_Torque_Down = 0;
          LLB_Pos_Up = 0;
          LLB_Pos_Down = 0;
          LLW_Freq = 0;
          LLW_Torque_Up = 0;
          LLW_Torque_Down = 0;
          LLW_Pos_Up = 0;
          LLW_Pos_Down = 0;
          Freq_Up_temp = 0;
          Freq_Down_temp = 0;
        state Freq_Up
          if(Freq_Up==0)
          Freq_Up_temp = 0;
          LLW_Freq = 1;
          end
        state Freq_Down
          if(Freq_Down==0)
          Freq_Down_temp = 0;
          LLW_Freq = -1;
          end
        (default) -> Adjust.LLW_Adjust.LLW_Freq_Adjust.LLW_Freq_Adjust
        Adjust.LLW_Adjust.LLW_Freq_Adjust.LLW_Freq_Adjust -> Adjust.LLW_Adjust.LLW_Freq_Adjust.Freq_Down [order 2] : [(Freq_Down_temp==0)&&(Freq_Down>0)]{Freq_Down_temp=1;}
        Adjust.LLW_Adjust.LLW_Freq_Adjust.LLW_Freq_Adjust -> Adjust.LLW_Adjust.LLW_Freq_Adjust.Freq_Up [order 1] : [(Freq_Up_temp==0)&&(Freq_Up>0)]{Freq_Up_temp=1;}
        Adjust.LLW_Adjust.LLW_Freq_Adjust.Freq_Up -> Adjust.LLW_Adjust.LLW_Freq_Adjust.LLW_Freq_Adjust : [Freq_Up_temp == 0]
        Adjust.LLW_Adjust.LLW_Freq_Adjust.Freq_Down -> Adjust.LLW_Adjust.LLW_Freq_Adjust.LLW_Freq_Adjust : [Freq_Down_temp == 0]
      state LLW_Torque_Adjust
        state Negtive_Up
          if(Negtive_Up==0)
          Negtive_Up_temp = 0;
          LLW_Torque_Down = 1;
          end
        state LLW_Torque_Adjust
          kState = "LLW_Torq";
          LLFK_Freq = 0;
          LLFK_Torque_Up = 0;
          LLFK_Torque_Down = 0;
          LLFK_Pos_Up = 0;
          LLFK_Pos_Down = 0;
          LLB_Freq = 0;
          LLB_Torque_Up = 0;
          LLB_Torque_Down = 0;
          LLB_Pos_Up = 0;
          LLB_Pos_Down = 0;
          LLW_Freq = 0;
          LLW_Torque_Up = 0;
          LLW_Torque_Down = 0;
          LLW_Pos_Up = 0;
          LLW_Pos_Down = 0;
          Negtive_Up_temp = 0;
          Negtive_Down_temp = 0;
          Positive_Up_temp = 0;
          Positive_Down_temp = 0;
        state Negtive_Down
          if(Negtive_Down==0)
          Negtive_Down_temp = 0;
          LLW_Torque_Down = -1;
          end
        state Positive_Up
          if(Positive_Up==0)
          Positive_Up_temp = 0;
          LLW_Torque_Up = 1;
          end
        state Positive_Down
          if(Positive_Down==0)
          Positive_Down_temp = 0;
          LLW_Torque_Up = -1;
          end
        (default) -> Adjust.LLW_Adjust.LLW_Torque_Adjust.LLW_Torque_Adjust
        Adjust.LLW_Adjust.LLW_Torque_Adjust.LLW_Torque_Adjust -> Adjust.LLW_Adjust.LLW_Torque_Adjust.Negtive_Up [order 4] : [(Negtive_Up_temp==0)&&(Negtive_Up>0)]{Negtive_Up_temp=1;}
        Adjust.LLW_Adjust.LLW_Torque_Adjust.LLW_Torque_Adjust -> Adjust.LLW_Adjust.LLW_Torque_Adjust.Negtive_Down [order 2] : [(Negtive_Down_temp==0)&&(Negtive_Down>0)]{Negtive_Down_temp=1;}
        Adjust.LLW_Adjust.LLW_Torque_Adjust.Negtive_Down -> Adjust.LLW_Adjust.LLW_Torque_Adjust.LLW_Torque_Adjust : [Negtive_Down_temp == 0]
        Adjust.LLW_Adjust.LLW_Torque_Adjust.Negtive_Up -> Adjust.LLW_Adjust.LLW_Torque_Adjust.LLW_Torque_Adjust : [Negtive_Up_temp == 0]
        Adjust.LLW_Adjust.LLW_Torque_Adjust.LLW_Torque_Adjust -> Adjust.LLW_Adjust.LLW_Torque_Adjust.Positive_Down [order 1] : [(Positive_Down_temp==0)&&(Positive_Down>0)]{Positive_Down_temp=1;}
        Adjust.LLW_Adjust.LLW_Torque_Adjust.LLW_Torque_Adjust -> Adjust.LLW_Adjust.LLW_Torque_Adjust.Positive_Up [order 3] : [(Positive_Up_temp==0)&&(Positive_Up>0)]{Positive_Up_temp=1;}
        Adjust.LLW_Adjust.LLW_Torque_Adjust.Positive_Up -> Adjust.LLW_Adjust.LLW_Torque_Adjust.LLW_Torque_Adjust : [Positive_Up_temp == 0]
        Adjust.LLW_Adjust.LLW_Torque_Adjust.Positive_Down -> Adjust.LLW_Adjust.LLW_Torque_Adjust.LLW_Torque_Adjust : [Positive_Down_temp == 0]
      state LLW_Pos_Adjust
        state Negtive_Up
          if(Negtive_Up==0)
          Negtive_Up_temp = 0;
          LLW_Pos_Down = 1;
          end
        state LLW_Pos_Adjust
          kState = "LLW_Pos";
          LLFK_Freq = 0;
          LLFK_Torque_Up = 0;
          LLFK_Torque_Down = 0;
          LLFK_Pos_Up = 0;
          LLFK_Pos_Down = 0;
          LLB_Freq = 0;
          LLB_Torque_Up = 0;
          LLB_Torque_Down = 0;
          LLB_Pos_Up = 0;
          LLB_Pos_Down = 0;
          LLW_Freq = 0;
          LLW_Torque_Up = 0;
          LLW_Torque_Down = 0;
          LLW_Pos_Up = 0;
          LLW_Pos_Down = 0;
          Negtive_Up_temp = 0;
          Negtive_Down_temp = 0;
          Positive_Up_temp = 0;
          Positive_Down_temp = 0;
        state Negtive_Down
          if(Negtive_Down==0)
          Negtive_Down_temp = 0;
          LLW_Pos_Down = -1;
          end
        state Positive_Up
          if(Positive_Up==0)
          Positive_Up_temp = 0;
          LLW_Pos_Up = 1;
          end
        state Positive_Down
          if(Positive_Down==0)
          Positive_Down_temp = 0;
          LLW_Pos_Up = -1;
          end
        (default) -> Adjust.LLW_Adjust.LLW_Pos_Adjust.LLW_Pos_Adjust
        Adjust.LLW_Adjust.LLW_Pos_Adjust.LLW_Pos_Adjust -> Adjust.LLW_Adjust.LLW_Pos_Adjust.Negtive_Up [order 4] : [(Negtive_Up_temp==0)&&(Negtive_Up>0)]{Negtive_Up_temp=1;}
        Adjust.LLW_Adjust.LLW_Pos_Adjust.LLW_Pos_Adjust -> Adjust.LLW_Adjust.LLW_Pos_Adjust.Negtive_Down [order 2] : [(Negtive_Down_temp==0)&&(Negtive_Down>0)]{Negtive_Down_temp=1;}
        Adjust.LLW_Adjust.LLW_Pos_Adjust.Negtive_Down -> Adjust.LLW_Adjust.LLW_Pos_Adjust.LLW_Pos_Adjust : [Negtive_Down_temp == 0]
        Adjust.LLW_Adjust.LLW_Pos_Adjust.Negtive_Up -> Adjust.LLW_Adjust.LLW_Pos_Adjust.LLW_Pos_Adjust : [Negtive_Up_temp == 0]
        Adjust.LLW_Adjust.LLW_Pos_Adjust.LLW_Pos_Adjust -> Adjust.LLW_Adjust.LLW_Pos_Adjust.Positive_Up [order 3] : [(Positive_Up_temp==0)&&(Positive_Up>0)]{Positive_Up_temp=1;}
        Adjust.LLW_Adjust.LLW_Pos_Adjust.LLW_Pos_Adjust -> Adjust.LLW_Adjust.LLW_Pos_Adjust.Positive_Down [order 1] : [(Positive_Down_temp==0)&&(Positive_Down>0)]{Positive_Down_temp=1;}
        Adjust.LLW_Adjust.LLW_Pos_Adjust.Positive_Up -> Adjust.LLW_Adjust.LLW_Pos_Adjust.LLW_Pos_Adjust : [Positive_Up_temp == 0]
        Adjust.LLW_Adjust.LLW_Pos_Adjust.Positive_Down -> Adjust.LLW_Adjust.LLW_Pos_Adjust.LLW_Pos_Adjust : [Positive_Down_temp == 0]
      Adjust.LLW_Adjust.LLW_Adjust -> LLW_Auto [order 4] : [ManualAuto=="LLW_Auto"]{Display_State=1;}
      LLW_Auto -> Adjust.LLW_Adjust.LLW_Adjust : [ManualAuto~="LLW_Auto"]{Display_State=4;}
      (default) -> Adjust.LLW_Adjust.LLW_Adjust
      Adjust.LLW_Adjust.LLW_Adjust -> Adjust.LLW_Adjust.LLW_Pos_Adjust [order 1] : [ManualAuto=="LLW_Manual_Pos"]
      Adjust.LLW_Adjust.LLW_Adjust -> Adjust.LLW_Adjust.LLW_Freq_Adjust [order 3] : [ManualAuto=="LLW_Manual_Freq"]
      Adjust.LLW_Adjust.LLW_Pos_Adjust -> Adjust.LLW_Adjust.LLW_Adjust : [ManualAuto~="LLW_Manual_Pos"]
      Adjust.LLW_Adjust.LLW_Freq_Adjust -> Adjust.LLW_Adjust.LLW_Adjust : [ManualAuto~="LLW_Manual_Freq"]
      Adjust.LLW_Adjust.LLW_Adjust -> Adjust.LLW_Adjust.LLW_Torque_Adjust [order 2] : [ManualAuto=="LLW_Manual_Torque"]
      Adjust.LLW_Adjust.LLW_Torque_Adjust -> Adjust.LLW_Adjust.LLW_Adjust : [ManualAuto~="LLW_Manual_Torque"]
    Adjust.Adjust -> LLF_Adjust [order 4] : [Mode=="Lower_Limb_Follow"]{Display_State=1;}
    LLF_Adjust -> Adjust.Adjust : [Mode~="Lower_Limb_Follow"]
    (default) -> Adjust.Adjust
    Adjust.Adjust -> Adjust.LLW_Adjust [order 1] : [Mode=="Lower_Limb_Walk"]{Display_State=4;}
    Adjust.Adjust -> Adjust.LLFK_Adjust [order 2] : [Mode=="Lower_Limb_FlutterKick"]{Display_State=2;}
    Adjust.LLW_Adjust -> Adjust.Adjust : [Mode~="Lower_Limb_Walk"]
    Adjust.LLFK_Adjust -> Adjust.Adjust : [Mode~="Lower_Limb_FlutterKick"]
    Adjust.LLB_Adjust -> Adjust.Adjust : [Mode~="Lower_Limb_Breaststroke"]
    Adjust.Adjust -> Adjust.LLB_Adjust [order 3] : [Mode=="Lower_Limb_Breaststroke"]{Display_State=3;}
  (default) -> Start
  Start -> Adjust : [State == "Stop"]
  Adjust -> Start : [State ~= "Stop"]
  data: kState output string; Display_State output; Freq_Up input; Freq_Down input; Positive_Up input; Positive_Down input; Negtive_Up input; Negtive_Down input; LLFK_Torque_Up output; LLFK_Torque_Down output; LLFK_Freq output; LLFK_Pos_Up output; LLFK_Pos_Down output; State input; Mode input; ManualAuto input; LLB_Freq output; LLB_Torque_Up output; LLB_Torque_Down output; LLB_Pos_Up output; LLB_Pos_Down output; LLW_Freq output; LLW_Torque_Up output; LLW_Torque_Down output; LLW_Pos_Up output; LLW_Pos_Down output; Freq_Up_temp local; Freq_Down_temp local; Positive_Up_temp local; Negtive_Up_temp local; Positive_Down_temp local; Negtive_Down_temp local

== matlab function PannelTest/Tasks/StopTask/MATLAB Function2 ==
  data: u input; y output; Pos input
function y = Current_P(u, Pos)
y = sign(u)*min(abs(u),abs(Pos)*0.1);

== matlab function PannelTest/Tasks/StopTask/MATLAB Function3 ==
  data: u input; y output; Pos input
function y = Current_P(u, Pos)
y = sign(u)*min(abs(u),abs(Pos)*0.1);
